simulink model "duc_cosim"  (Simulink 7.7)
settings: Solver=FixedStepDiscrete  SolverMode=SingleTasking  StartTime=0.0  StopTime=.01  FixedStep=1e-7  RelTol=1e-3
libraries: modelsimlib x1
settings Model: Creator=embed  LastModifiedBy=embed
settings SolverCC: AutoInsertRateTranBlk=on

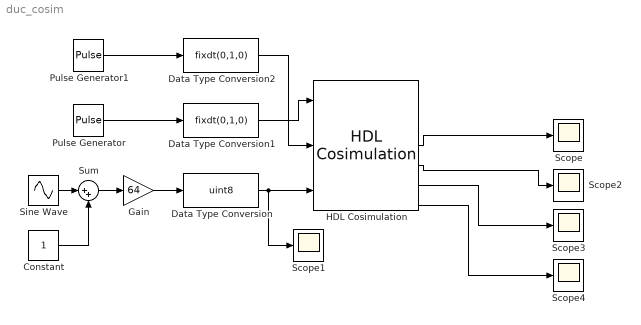
== system duc_cosim ==
  Constant : Constant
  Data Type Conversion : DataTypeConversion  OutDataTypeStr=uint8
  Data Type Conversion1 : DataTypeConversion  OutDataTypeStr=fixdt(0,1,0)
  Data Type Conversion2 : DataTypeConversion  OutDataTypeStr=fixdt(0,1,0)
  Gain : Gain  Gain=64
  HDL Cosimulation : modelsimlib/HDL Cosimulation  SystemSampleTime=-1  PortPaths=/top/clk;/top/clk_out;/top/ctl0;/top/rdy;/top/clk_out1;/top/data_in;/top/data_out;/top/po;/top/co;/top/dds1/cosine  PortModes=[1 2 1 2 2 1 2 2 2 2 ]  PortTimes=[-1,1e-7,-1,1e-7,1e-7,-1,1e-7,1e-7,1e-7,1e-7]  PortSigns=[-1 -1 -1 -1 -1 -1 1 1 1 1 ]  PortFracLengths=[0,0,0,0,0,0,0,0,0,0]  CommLocal=on  CommSharedMemory=off  CommPortNumber=4449  CommShowInfo=on  ClockPaths=/top/clk  ClockModes=[2 ]  ClockTimes=[1]  TclPreSimCommand="puts \"Running Simulink Cosimulation block.\""  TclPostSimCommand="puts \"done\""  TimingMode=Tick  TimingScaleFactor=10e6  idxCellArray={'UNUSED_VAR'}  CosimBypass=Full Simulation  AllowDirectFeedthrough=off  ProductName=EDA Simulator Link MQ  RunAutoTimescale=off  HdlClocks=0
  Pulse Generator : DiscretePulseGenerator  SampleTime=1e-7
  Pulse Generator1 : DiscretePulseGenerator  SampleTime=512/10e6
  Scope{,1..4} (5 alike) : Scope
      Scope settings: YMin=-70  YMax=60  MaxDataPoints=100000
      Scope1 settings: YMin=0  YMax=275
      Scope2 settings: YMin=-17500  YMax=17500  SaveName=ScopeData2  MaxDataPoints=100000
      Scope3 settings: YMin=-150  YMax=125  SaveName=ScopeData3  MaxDataPoints=100000
      Scope4 settings: YMin=-150  YMax=150  SaveName=ScopeData4  MaxDataPoints=100000
  Sine Wave : Sin  SineType=Sample based  Samples=195  SampleTime=512/10e6
  Sum : Sum  Inputs=|++
  wires:
  HDL Cosimulation/4 -> Scope/1
  Data Type Conversion/1 -> HDL Cosimulation/3, Scope1/1
  Gain/1 -> Data Type Conversion/1
  Sine Wave/1 -> Sum/1
  Sum/1 -> Gain/1
  Constant/1 -> Sum/2
  Pulse Generator/1 -> Data Type Conversion1/1
  Data Type Conversion1/1 -> HDL Cosimulation/1
  Pulse Generator1/1 -> Data Type Conversion2/1
  Data Type Conversion2/1 -> HDL Cosimulation/2
  HDL Cosimulation/5 -> Scope2/1
  HDL Cosimulation/6 -> Scope3/1
  HDL Cosimulation/7 -> Scope4/1
